simulink model "half_passive"  (Simulink 4.00)
settings: Solver=ode45  StartTime=0.0  StopTime=10.0  RelTol=1e-3
libraries: simulink3 x1
settings Model: LastModifiedBy=administrator

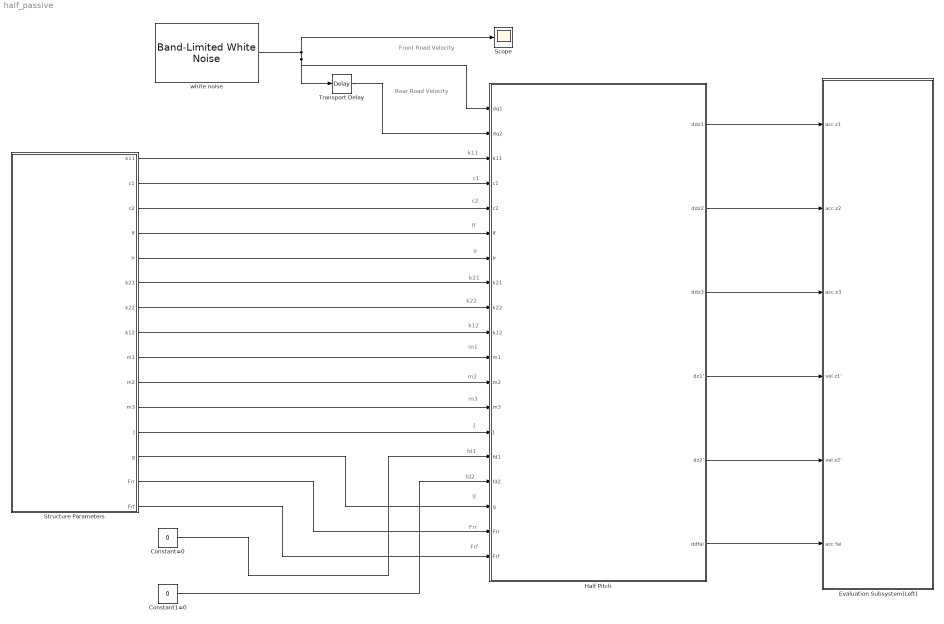
== system half_passive ==
  note: Front Road Velocity
  note: Rear Road Velocity
  note: c1
  note: lr
  note: lf
  note: m3
  note: m2
  note: m1
  note: k22
  note: k21
  note: k12
  note: k11
  note: c2
  note: J
  note: fd1
  note: fd2
  note: g
  note: Frr
  note: Frf
  " white noise" : simulink3/Sources/Band-Limited White Noise  Cov=[256*10^-6]  Ts=0.01  seed=[23341]
  Constant1=0 : Constant  Value=0
  Constant=0 : Constant  Value=0
  Evaluation Subsystem(Left) : Subsystem
      settings: RTWFcnNameOpts=Auto  RTWFileNameOpts=Auto
  Half Pitch : Subsystem
      settings: RTWFcnNameOpts=Auto  RTWFileNameOpts=Auto
      mask Display: disp('Half Pitch)')
  Scope : Scope
      settings: TimeRange=auto  YMin=-5  YMax=5  SaveToWorkspace=off  SaveName=ScopeData18  LimitDataPoints=on  MaxDataPoints=5000
  "Structure Parameters " : Subsystem
      settings: RTWFcnNameOpts=Auto  RTWFileNameOpts=Auto
  Transport Delay : TransportDelay  DelayTime=1  InitialInput=0  BufferSize=1024  PadeOrder=0
  wires:
  " white noise"/1 -> Transport Delay/1, Half Pitch/1(dq1), Scope/1
  Transport Delay/1 -> Half Pitch/2(dq2)
  "Structure Parameters "/1("k11 ") -> Half Pitch/3(k11)
  "Structure Parameters "/2(c1) -> Half Pitch/4(c1)
  "Structure Parameters "/3(c2) -> Half Pitch/5(c2)
  "Structure Parameters "/4(lf) -> Half Pitch/6(lf)
  "Structure Parameters "/5(lr) -> Half Pitch/7(lr)
  "Structure Parameters "/6(k21) -> Half Pitch/8(k21)
  "Structure Parameters "/7(k22) -> Half Pitch/9(k22)
  "Structure Parameters "/8(k12) -> Half Pitch/10(k12)
  "Structure Parameters "/9(m1) -> Half Pitch/11(m1)
  "Structure Parameters "/10(m2) -> Half Pitch/12(m2)
  "Structure Parameters "/11(m3) -> Half Pitch/13(m3)
  "Structure Parameters "/12(J) -> Half Pitch/14(J)
  "Structure Parameters "/15(Frf) -> Half Pitch/19(Frf)
  "Structure Parameters "/14(Frr) -> Half Pitch/18(Frr)
  "Structure Parameters "/13(g) -> Half Pitch/17(g)
  Constant=0/1 -> Half Pitch/15(fd1)
  Constant1=0/1 -> Half Pitch/16(fd2)
  Half Pitch/6(ddfai) -> Evaluation Subsystem(Left)/6(acc fai)
  Half Pitch/5(dz2') -> Evaluation Subsystem(Left)/5(vel z2')
  Half Pitch/4(dz1') -> Evaluation Subsystem(Left)/4(vel z1')
  Half Pitch/3(ddz3) -> Evaluation Subsystem(Left)/3(acc z3)
  Half Pitch/2(ddz2) -> Evaluation Subsystem(Left)/2(acc z2)
  Half Pitch/1(ddz1) -> Evaluation Subsystem(Left)/1(acc z1)

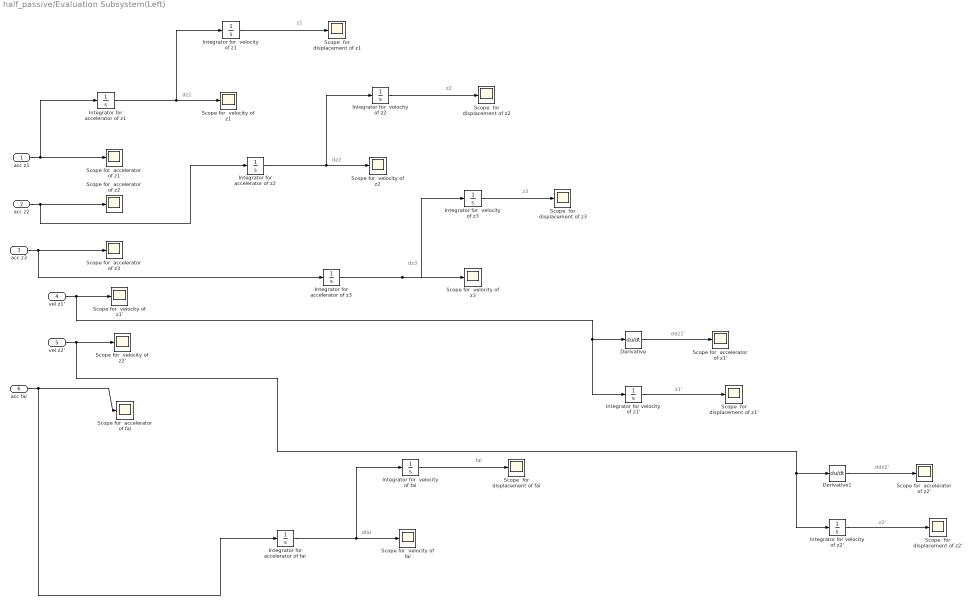
== system half_passive/Evaluation Subsystem(Left) ==
  note: dz1
  note: z1
  note: dz2
  note: z2
  note: dz3
  note: z3
  note: dfai
  note: fai
  note: ddz1'
  note: z1'
  note: ddz2'
  note: z2'
  acc z1 : Inport  Port=1  LatchInput=off
  acc z2 : Inport  Port=2  LatchInput=off
  acc z3 : Inport  Port=3  LatchInput=off
  vel z1' : Inport  Port=4  LatchInput=off
  vel z2' : Inport  Port=5  LatchInput=off
  acc fai : Inport  Port=6  LatchInput=off
  Derivative : Derivative
  Derivative1 : Derivative
  Integrator for accelerator of fai : Integrator  ExternalReset=none  InitialConditionSource=internal  InitialCondition=0  LimitOutput=off  UpperSaturationLimit=inf  LowerSaturationLimit=-inf  ShowSaturationPort=off  ShowStatePort=off  AbsoluteTolerance=auto
  Integrator for accelerator of z1 : Integrator  ExternalReset=none  InitialConditionSource=internal  InitialCondition=0  LimitOutput=off  UpperSaturationLimit=inf  LowerSaturationLimit=-inf  ShowSaturationPort=off  ShowStatePort=off  AbsoluteTolerance=auto
  Integrator for accelerator of z2 : Integrator  ExternalReset=none  InitialConditionSource=internal  InitialCondition=0  LimitOutput=off  UpperSaturationLimit=inf  LowerSaturationLimit=-inf  ShowSaturationPort=off  ShowStatePort=off  AbsoluteTolerance=auto
  Integrator for accelerator of z3 : Integrator  ExternalReset=none  InitialConditionSource=internal  InitialCondition=0  LimitOutput=off  UpperSaturationLimit=inf  LowerSaturationLimit=-inf  ShowSaturationPort=off  ShowStatePort=off  AbsoluteTolerance=auto
  Integrator for velocity of z1' : Integrator  ExternalReset=none  InitialConditionSource=internal  InitialCondition=0  LimitOutput=off  UpperSaturationLimit=inf  LowerSaturationLimit=-inf  ShowSaturationPort=off  ShowStatePort=off  AbsoluteTolerance=auto
  Integrator for velocity of z2' : Integrator  ExternalReset=none  InitialConditionSource=internal  InitialCondition=0  LimitOutput=off  UpperSaturationLimit=inf  LowerSaturationLimit=-inf  ShowSaturationPort=off  ShowStatePort=off  AbsoluteTolerance=auto
  Integrator for  velocity of fai : Integrator  ExternalReset=none  InitialConditionSource=internal  InitialCondition=0  LimitOutput=off  UpperSaturationLimit=inf  LowerSaturationLimit=-inf  ShowSaturationPort=off  ShowStatePort=off  AbsoluteTolerance=auto
  "Integrator for  velocity of z1 " : Integrator  ExternalReset=none  InitialConditionSource=internal  InitialCondition=0  LimitOutput=off  UpperSaturationLimit=inf  LowerSaturationLimit=-inf  ShowSaturationPort=off  ShowStatePort=off  AbsoluteTolerance=auto
  Integrator for  velocity of z2 : Integrator  ExternalReset=none  InitialConditionSource=internal  InitialCondition=0  LimitOutput=off  UpperSaturationLimit=inf  LowerSaturationLimit=-inf  ShowSaturationPort=off  ShowStatePort=off  AbsoluteTolerance=auto
  Integrator for  velocity of z3 : Integrator  ExternalReset=none  InitialConditionSource=internal  InitialCondition=0  LimitOutput=off  UpperSaturationLimit=inf  LowerSaturationLimit=-inf  ShowSaturationPort=off  ShowStatePort=off  AbsoluteTolerance=auto
  Scope  for displacement of fai : Scope
      settings: TimeRange=auto  YMin=-0.8  YMax=-0.2  SaveToWorkspace=off  SaveName=ScopeData12  LimitDataPoints=on  MaxDataPoints=5000
  "Scope  for displacement of z1  " : Scope
      settings: TimeRange=auto  YMin=28.5  YMax=33.5  SaveToWorkspace=off  SaveName=ScopeData5  LimitDataPoints=on  MaxDataPoints=5000
  Scope  for displacement of z1' : Scope
      settings: TimeRange=auto  YMin=3  YMax=8.5  SaveToWorkspace=off  SaveName=ScopeData15  LimitDataPoints=on  MaxDataPoints=5000
  Scope  for displacement of z2 : Scope
      settings: TimeRange=auto  YMin=5.5  YMax=8.5  SaveToWorkspace=off  SaveName=ScopeData8  LimitDataPoints=on  MaxDataPoints=5000
  Scope  for displacement of z2' : Scope
      settings: TimeRange=auto  YMin=-5  YMax=5  SaveToWorkspace=off  SaveName=ScopeData16  LimitDataPoints=on  MaxDataPoints=5000
  Scope  for displacement of z3 : Scope
      settings: TimeRange=auto  YMin=-39.9  YMax=-38.4  SaveToWorkspace=off  SaveName=ScopeData10  LimitDataPoints=on  MaxDataPoints=5000
  Scope for  accelerator of fai : Scope
      settings: TimeRange=10  YMin=-0.5  YMax=0.4  SaveToWorkspace=off  SaveName=ScopeData3  LimitDataPoints=on  MaxDataPoints=5000
  Scope for  accelerator of z1 : Scope
      settings: TimeRange=10  YMin=-0.8  YMax=0.6  SaveToWorkspace=off  SaveName=ScopeData  LimitDataPoints=on  MaxDataPoints=5000
  Scope for  accelerator of z1' : Scope
      settings: TimeRange=auto  YMin=-5  YMax=5  SaveToWorkspace=off  SaveName=ScopeData14  LimitDataPoints=on  MaxDataPoints=5000
  Scope for  accelerator of z2 : Scope
      settings: TimeRange=auto  YMin=-0.8  YMax=0.9  SaveToWorkspace=off  LimitDataPoints=on  MaxDataPoints=5000
  Scope for  accelerator of z2' : Scope
      settings: TimeRange=auto  YMin=-5  YMax=5  SaveToWorkspace=off  SaveName=ScopeData17  LimitDataPoints=on  MaxDataPoints=5000
  Scope for  accelerator of z3 : Scope
      settings: TimeRange=auto  YMin=-1  YMax=1.25  SaveToWorkspace=off  SaveName=ScopeData2  LimitDataPoints=on  MaxDataPoints=5000
  Scope for  velocity of fai : Scope
      settings: TimeRange=auto  YMin=-5  YMax=5  SaveToWorkspace=off  SaveName=ScopeData13  LimitDataPoints=on  MaxDataPoints=5000
  "Scope for  velocity of z1 " : Scope
      settings: TimeRange=auto  YMin=-5  YMax=5  SaveToWorkspace=off  SaveName=ScopeData7  LimitDataPoints=on  MaxDataPoints=5000
  Scope for  velocity of z1' : Scope
      settings: TimeRange=auto  YMin=-5  YMax=5  SaveToWorkspace=off  SaveName=ScopeData4  LimitDataPoints=on  MaxDataPoints=5000
  "Scope for  velocity of z2 " : Scope
      settings: TimeRange=auto  YMin=-5  YMax=5  SaveToWorkspace=off  SaveName=ScopeData9  LimitDataPoints=on  MaxDataPoints=5000
  Scope for  velocity of z2' : Scope
      settings: TimeRange=auto  YMin=-5  YMax=5  SaveToWorkspace=off  SaveName=ScopeData6  LimitDataPoints=on  MaxDataPoints=5000
  Scope for  velocity of z3 : Scope
      settings: TimeRange=auto  YMin=-5  YMax=5  SaveToWorkspace=off  SaveName=ScopeData11  LimitDataPoints=on  MaxDataPoints=5000
  wires:
  acc z1/1 -> Integrator for accelerator of z1/1, Scope for  accelerator of z1/1
  acc z2/1 -> Integrator for accelerator of z2/1, Scope for  accelerator of z2/1
  acc z3/1 -> Integrator for accelerator of z3/1, Scope for  accelerator of z3/1
  vel z1'/1 -> Integrator for velocity of z1'/1, Derivative/1, Scope for  velocity of z1'/1
  vel z2'/1 -> Integrator for velocity of z2'/1, Derivative1/1, Scope for  velocity of z2'/1
  acc fai/1 -> Integrator for accelerator of fai/1, Scope for  accelerator of fai/1
  Integrator for accelerator of z1/1 -> "Scope for  velocity of z1 "/1, "Integrator for  velocity of z1 "/1
  "Integrator for  velocity of z1 "/1 -> "Scope  for displacement of z1  "/1
  Integrator for accelerator of z2/1 -> "Scope for  velocity of z2 "/1, Integrator for  velocity of z2/1
  Integrator for  velocity of z2/1 -> Scope  for displacement of z2/1
  Integrator for accelerator of z3/1 -> Scope for  velocity of z3/1, Integrator for  velocity of z3/1
  Integrator for  velocity of z3/1 -> Scope  for displacement of z3/1
  Integrator for accelerator of fai/1 -> Scope for  velocity of fai/1, Integrator for  velocity of fai/1
  Integrator for  velocity of fai/1 -> Scope  for displacement of fai/1
  Derivative/1 -> Scope for  accelerator of z1'/1
  Integrator for velocity of z1'/1 -> Scope  for displacement of z1'/1
  Derivative1/1 -> Scope for  accelerator of z2'/1
  Integrator for velocity of z2'/1 -> Scope  for displacement of z2'/1

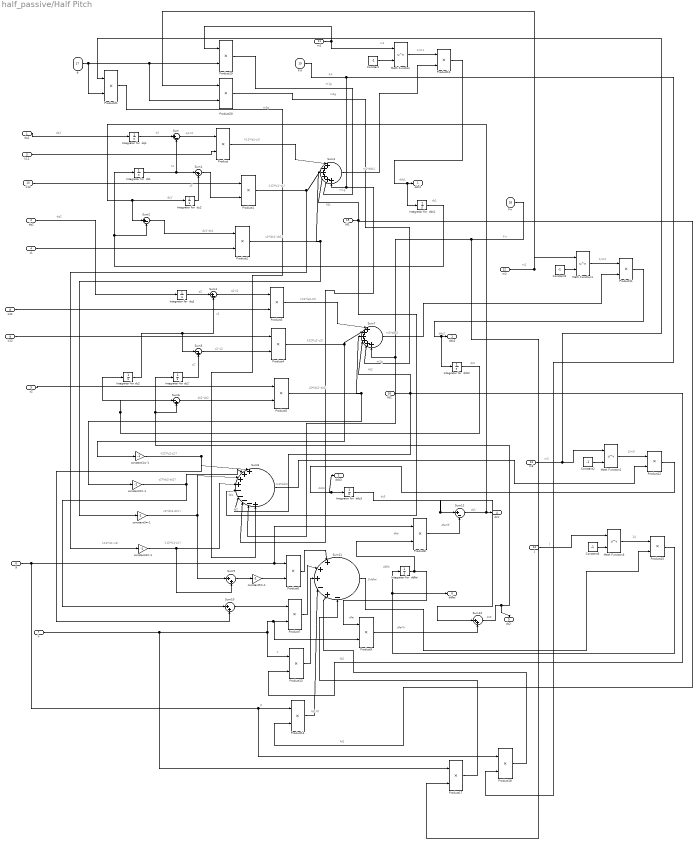
== system half_passive/Half Pitch ==
  note: dz2'
  note: dfai*lr
  note: dz1'
  note: dfai*lf
  note: dfai
  note: dfai
  note: ddfai
  note: J*ddfai
  note: dz3
  note: ddz3
  note: m3*ddz3
  note: c2*(dz2-dz2')
  note: c1*(dz1-dz1')
  note: k22*(z2-z2')
  note: k12*(z1-z1')
  note: k12*(z1'-z1)
  note: dz2
  note: ddz2
  note: m2*ddz2
  note: dz2'-dz2
  note: c2*(dz2'-dz2)
  note: k22*(z2'-z2)
  note: z2'-z2
  note: z2'
  note: k21*(q2-z2)
  note: q2-z2
  note: z2
  note: dz1
  note: ddz1
  note: m1*ddz1
  note: c1*(dz1'-dz1)
  note: dz1'-dz1
  note: dz1'
  note: k12*(z1'-z1)
  note: z1'
  note: k11*(q1-z1)
  note: q2
  note: q1-z1
  note: z1
  note: q1
  note: dq1
  note: dq2
  note: m1
  note: 1/m1
  note: m2
  note: 1/m2
  note: m3
  note: 1/m3
  note: fd1
  note: fd2
  note: fd1
  note: fd2
  note: fd2
  note: fd1
  note: lf
  note: fd1*lf
  note: lr
  note: J
  note: 1/J
  note: m1g
  note: m2g
  note: Frf
  note: Frr
  note: m3g
  note: m1g
  note: m2g
  dq1 : Inport  Port=1  LatchInput=off
  dq2 : Inport  Port=2  LatchInput=off
  k11 : Inport  Port=3  LatchInput=off
  c1 : Inport  Port=4  LatchInput=off
  c2 : Inport  Port=5  LatchInput=off
  lf : Inport  Port=6  LatchInput=off
  lr : Inport  Port=7  LatchInput=off
  k21 : Inport  Port=8  LatchInput=off
  k22 : Inport  Port=9  LatchInput=off
  k12 : Inport  Port=10  LatchInput=off
  m1 : Inport  Port=11  LatchInput=off
  m2 : Inport  Port=12  LatchInput=off
  m3 : Inport  Port=13  LatchInput=off
  J : Inport  Port=14  LatchInput=off
  fd1 : Inport  Port=15  LatchInput=off
  fd2 : Inport  Port=16  LatchInput=off
  g : Inport  Port=17  LatchInput=off
  Frr : Inport  Port=18  LatchInput=off
  Frf : Inport  Port=19  LatchInput=off
  Constant{,1..3} (4 alike) : Constant  Value=-1
  Integrator for  dq2 : Integrator  ExternalReset=none  InitialConditionSource=internal  InitialCondition=0  LimitOutput=off  UpperSaturationLimit=inf  LowerSaturationLimit=-inf  ShowSaturationPort=off  ShowStatePort=off  AbsoluteTolerance=auto
  Integrator for dz2 : Integrator  ExternalReset=none  InitialConditionSource=internal  InitialCondition=0  LimitOutput=off  UpperSaturationLimit=inf  LowerSaturationLimit=-inf  ShowSaturationPort=off  ShowStatePort=off  AbsoluteTolerance=auto
  Integrator for dz2' : Integrator  ExternalReset=none  InitialConditionSource=internal  InitialCondition=0  LimitOutput=off  UpperSaturationLimit=inf  LowerSaturationLimit=-inf  ShowSaturationPort=off  ShowStatePort=off  AbsoluteTolerance=auto
  Integrator for  ddfai : Integrator  ExternalReset=none  InitialConditionSource=internal  InitialCondition=0  LimitOutput=off  UpperSaturationLimit=inf  LowerSaturationLimit=-inf  ShowSaturationPort=off  ShowStatePort=off  AbsoluteTolerance=auto
  Integrator for  ddz1 : Integrator  ExternalReset=none  InitialConditionSource=internal  InitialCondition=0  LimitOutput=off  UpperSaturationLimit=inf  LowerSaturationLimit=-inf  ShowSaturationPort=off  ShowStatePort=off  AbsoluteTolerance=auto
  Integrator for  ddz2 : Integrator  ExternalReset=none  InitialConditionSource=internal  InitialCondition=0  LimitOutput=off  UpperSaturationLimit=inf  LowerSaturationLimit=-inf  ShowSaturationPort=off  ShowStatePort=off  AbsoluteTolerance=auto
  Integrator for  ddz3 : Integrator  ExternalReset=none  InitialConditionSource=internal  InitialCondition=0  LimitOutput=off  UpperSaturationLimit=inf  LowerSaturationLimit=-inf  ShowSaturationPort=off  ShowStatePort=off  AbsoluteTolerance=auto
  Integrator for  dq1 : Integrator  ExternalReset=none  InitialConditionSource=internal  InitialCondition=0  LimitOutput=off  UpperSaturationLimit=inf  LowerSaturationLimit=-inf  ShowSaturationPort=off  ShowStatePort=off  AbsoluteTolerance=auto
  Integrator for  dz1 : Integrator  ExternalReset=none  InitialConditionSource=internal  InitialCondition=0  LimitOutput=off  UpperSaturationLimit=inf  LowerSaturationLimit=-inf  ShowSaturationPort=off  ShowStatePort=off  AbsoluteTolerance=auto
  Integrator for  dz1' : Integrator  ExternalReset=none  InitialConditionSource=internal  InitialCondition=0  LimitOutput=off  UpperSaturationLimit=inf  LowerSaturationLimit=-inf  ShowSaturationPort=off  ShowStatePort=off  AbsoluteTolerance=auto
  Math Function{,1..3} (4 alike) : Math  Operator=pow  OutputSignalType=auto
  Product{,1..15,17..21} (21 alike) : Product  Inputs=2  Multiplication=Element-wise(.*)  SaturateOnIntegerOverflow=on
  Sum{,2,4,12} (4 alike) : Sum  Inputs=|+-  SaturateOnIntegerOverflow=on
  Sum1 : Sum  Inputs=|-+  SaturateOnIntegerOverflow=on
  Sum10 : Sum  Inputs=|++  SaturateOnIntegerOverflow=on
  Sum11 : Sum  Inputs=|+++-+-  SaturateOnIntegerOverflow=on
  Sum13 : Sum  Inputs=|++  SaturateOnIntegerOverflow=on
  Sum3 : Sum  Inputs=|++++++  SaturateOnIntegerOverflow=on
  Sum5 : Sum  Inputs=|-+  SaturateOnIntegerOverflow=on
  Sum6 : Sum  Inputs=|-+  SaturateOnIntegerOverflow=on
  Sum7 : Sum  Inputs=|++++++  SaturateOnIntegerOverflow=on
  Sum8 : Sum  Inputs=|++++----+  SaturateOnIntegerOverflow=on
  Sum9 : Sum  Inputs=|++  SaturateOnIntegerOverflow=on
  constant1=-1 : Gain  Gain=-1  Multiplication=Element-wise(K.*u)  SaturateOnIntegerOverflow=on
  constant2=-1 : Gain  Gain=-1  Multiplication=Element-wise(K.*u)  SaturateOnIntegerOverflow=on
  constant3=-1 : Gain  Gain=-1  Multiplication=Element-wise(K.*u)  SaturateOnIntegerOverflow=on
  constant4=-1 : Gain  Gain=-1  Multiplication=Element-wise(K.*u)  SaturateOnIntegerOverflow=on
  constant5=-1 : Gain  Gain=-1  Multiplication=Element-wise(K.*u)  SaturateOnIntegerOverflow=on
  ddz1 : Outport  Port=1
  ddz2 : Outport  Port=2
  ddz3 : Outport  Port=3
  dz1' : Outport  Port=4
  dz2' : Outport  Orientation=down  Port=5
  ddfai : Outport  Port=6
  wires:
  Sum13/1 -> Integrator for dz2'/1, Sum6/2, dz2'/1
  Product9/1 -> Sum13/2
  Sum12/1 -> Integrator for  dz1'/1, Sum2/1, dz1'/1
  Product8/1 -> Sum12/2
  Integrator for  ddfai/1 -> Product8/2, Product9/1
  Sum11/1 -> Product15/2
  Product7/1 -> Sum11/2
  Sum10/1 -> Product7/1
  lr/1 -> Product7/2, Product9/2, Product13/1, Product17/1
  Product6/1 -> Sum11/1
  constant5=-1/1 -> Product6/2
  Sum9/1 -> constant5=-1/1
  lf/1 -> Product6/1, Product8/1, Product14/1, Product18/1
  Integrator for  ddz3/1 -> Sum12/1, Sum13/1
  Sum8/1 -> Product12/2
  constant2=-1/1 -> Sum8/2, Sum10/1
  constant3=-1/1 -> Sum8/3, Sum9/1
  constant1=-1/1 -> Sum8/1, Sum10/2
  constant4=-1/1 -> Sum8/4, Sum9/2
  Integrator for  ddz2/1 -> Integrator for dz2/1, Sum6/1
  Sum7/1 -> Product11/2
  Product5/1 -> Sum7/3, constant2=-1/1
  Sum6/1 -> Product5/2
  c2/1 -> Product5/1
  Product4/1 -> Sum7/2, constant1=-1/1
  Sum5/1 -> Product4/2
  Integrator for dz2'/1 -> Sum5/2
  k22/1 -> Product4/1
  Product3/1 -> Sum7/1
  k21/1 -> Product3/2
  Sum4/1 -> Product3/1
  Integrator for dz2/1 -> Sum4/2, Sum5/1
  Integrator for  ddz1/1 -> Integrator for  dz1/1, Sum2/2
  Sum3/1 -> Product10/2
  Product2/1 -> Sum3/3, constant3=-1/1
  Sum2/1 -> Product2/1
  c1/1 -> Product2/2
  Product1/1 -> Sum3/2, constant4=-1/1
  Sum1/1 -> Product1/2
  k12/1 -> Product1/1
  Integrator for  dz1'/1 -> Sum1/2
  Product/1 -> Sum3/1
  k11/1 -> Product/2
  Integrator for  dq2/1 -> Sum4/1
  Sum/1 -> Product/1
  Integrator for  dq1/1 -> Sum/1
  Integrator for  dz1/1 -> Sum/2, Sum1/1
  dq2/1 -> Integrator for  dq2/1
  dq1/1 -> Integrator for  dq1/1
  Constant/1 -> Math Function/2
  m1/1 -> Product19/1, Math Function/1
  Math Function/1 -> Product10/1
  Product10/1 -> Integrator for  ddz1/1, ddz1/1
  Constant1/1 -> Math Function1/2
  m2/1 -> Product20/1, Math Function1/1
  Math Function1/1 -> Product11/1
  Product11/1 -> Integrator for  ddz2/1, ddz2/1
  Constant2/1 -> Math Function2/2
  m3/1 -> Product21/1, Math Function2/1
  Math Function2/1 -> Product12/1
  Product12/1 -> ddz3/1, Integrator for  ddz3/1
  fd1/1 -> Sum3/4, Product14/2, Sum8/5
  fd2/1 -> Sum7/4, Product13/2, Sum8/6
  Product13/1 -> Sum11/3
  Product14/1 -> Sum11/4
  Constant3/1 -> Math Function3/2
  J/1 -> Math Function3/1
  Math Function3/1 -> Product15/1
  Product15/1 -> Integrator for  ddfai/1, ddfai/1
  Frr/1 -> Sum7/6, Sum8/8, Product17/2
  Product17/1 -> Sum11/6
  Product18/1 -> Sum11/5
  g/1 -> Product19/2, Product20/2, Product21/2
  Product19/1 -> Sum3/5
  Product20/1 -> Sum7/5
  Product21/1 -> Sum8/9
  Frf/1 -> Sum3/6, Sum8/7, Product18/2

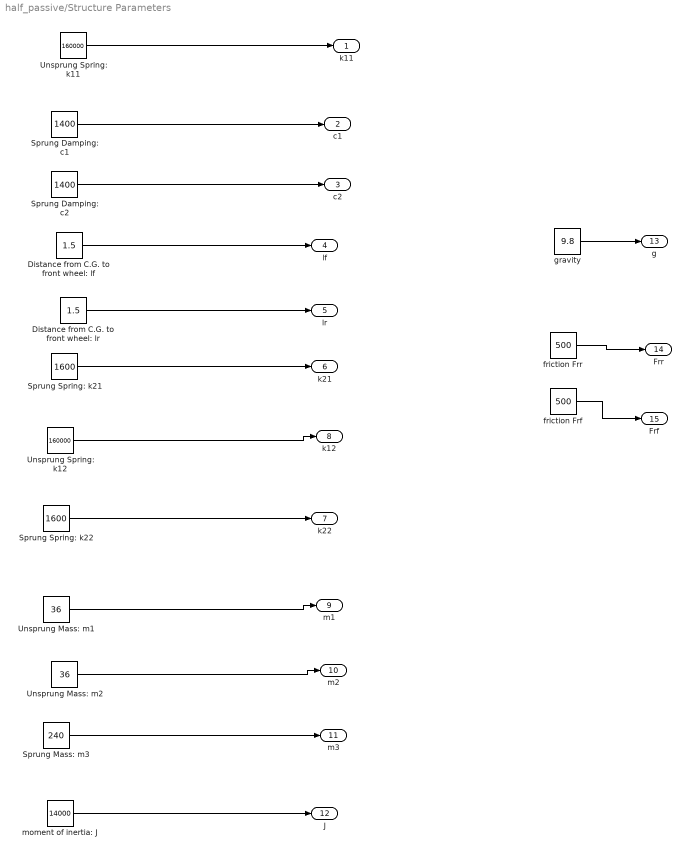
== system half_passive/Structure Parameters  ==
  " Sprung Damping: c1" : Constant  Value=1400
  " Sprung Damping: c2" : Constant  Value=1400
  " Sprung Spring: k21" : Constant  Value=1600
  " Sprung Spring: k22" : Constant  Value=1600
  Distance from C.G. to front wheel: lf : Constant  Value=1.5
  Distance from C.G. to front wheel: lr : Constant  Value=1.5
  Sprung Mass: m3 : Constant  Value=240
  Unsprung Mass: m1 : Constant  Value=36
  Unsprung Mass: m2 : Constant  Value=36
  Unsprung Spring: k11 : Constant  Value=160000
  Unsprung Spring: k12 : Constant  Value=160000
  friction Frf : Constant  Value=500
  friction Frr : Constant  Value=500
  gravity : Constant  Value=9.8
  moment of inertia: J : Constant  Value=14000
  "k11 " : Outport  Port=1
  c1 : Outport  Port=2
  c2 : Outport  Port=3
  lf : Outport  Port=4
  lr : Outport  Port=5
  k21 : Outport  Port=6
  k22 : Outport  Port=7
  k12 : Outport  Port=8
  m1 : Outport  Port=9
  m2 : Outport  Port=10
  m3 : Outport  Port=11
  J : Outport  Port=12
  g : Outport  Port=13
  Frr : Outport  Port=14
  Frf : Outport  Port=15
  wires:
  Unsprung Spring: k11/1 -> "k11 "/1
  " Sprung Damping: c1"/1 -> c1/1
  " Sprung Damping: c2"/1 -> c2/1
  Distance from C.G. to front wheel: lf/1 -> lf/1
  Distance from C.G. to front wheel: lr/1 -> lr/1
  " Sprung Spring: k21"/1 -> k21/1
  Unsprung Spring: k12/1 -> k12/1
  " Sprung Spring: k22"/1 -> k22/1
  Unsprung Mass: m1/1 -> m1/1
  Unsprung Mass: m2/1 -> m2/1
  Sprung Mass: m3/1 -> m3/1
  moment of inertia: J/1 -> J/1
  gravity/1 -> g/1
  friction Frr/1 -> Frr/1
  friction Frf/1 -> Frf/1
